simulink model "dcdctest"  (R2023b)
settings: Solver=VariableStepAuto  StartTime=0.0  StopTime=10  RelTol=1e-3
values from neighbouring files (symbols this model uses):
  cell_cap_Ah = 2.2    [find_maximum_ovlp.m]    (also in main.m)
  dst_q_cls = zeros(50, 2)    [main.m]
  dst_trg_soc_av = zeros(50, 1)    [main.m]
  soc = soc_in    [balance_costF.m]    (also in find_maximum_ovlp.m = fix(rand (1, cell_count) * 100); log_clustering.m; main.m = [39    39    20    72    81    92    51    11    60]; plot_final.m)
  src_q_cls = zeros(50, 2)    [main.m]
  src_trg_soc_av = zeros(50, 1)    [main.m]
undefined symbols (not defined in the file or in its folder): Ion, Lithium
libraries: spsIdealSwitchLib x18, spsBatteryLib x12, spsControlledCurrentSourceLib x8, spsVoltageMeasurementLib x8, simulink x4, slpidlib x3, spspowerguiLib x2
(part 2 of 2)

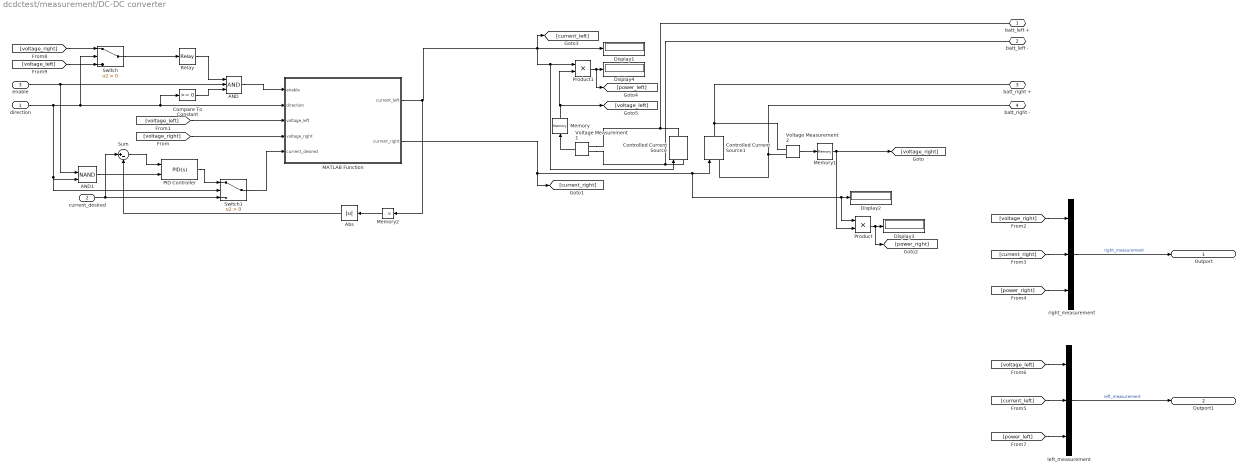
== system dcdctest/measurement/DC-DC converter ==
  direction : Inport
  current_desired : Inport  Port=2
  enable : Inport  Port=3
  AND : Logic  Inputs=3  IconShape=distinctive  AllPortsSameDT=off  OutDataTypeStr=boolean
  AND1 : Logic  Operator=NAND  IconShape=distinctive  AllPortsSameDT=off  OutDataTypeStr=boolean
  Abs : Abs  SaturateOnIntegerOverflow=off
  Compare To Constant : simulink/Logic and Bit Operations/Compare To Constant  relop=>=  const=0  OutDataTypeStr=boolean
  Controlled Current Source : spsControlledCurrentSourceLib/Controlled Current Source  Initialize=on  Source_Type=DC  Amplitude=0  Phase=0  Frequency=0  Measurements=None
  Controlled Current Source1 : spsControlledCurrentSourceLib/Controlled Current Source  Initialize=on  Source_Type=AC  Amplitude=0  Phase=0  Frequency=0  Measurements=None
  Display{1..4} (4 alike) : Display
  MATLAB Function : MATLAB Function  TreatAsAtomicUnit=on
  Memory : Memory
  Memory1 : Memory
  Memory2 : Memory
  PID Controller : slpidlib/PID Controller  Controller=PID  Form=Parallel  TimeDomain=Continuous-time  UseExternalTs=off  SampleTime=-1  IntegratorMethod=Forward Euler  FilterMethod=Forward Euler  ControllerParametersSource=internal  P=0.01  I=2  UseKiTs=off  D=0  N=100  UseFilter=on  TunerSelectOption=Transfer Function Based (PID Tuner App)  InitialConditionSource=internal  InitialConditionForIntegrator=0  InitialConditionForFilter=0  DifferentiatorICPrevScaledInput=0  ExternalReset=level  TrackingMode=off  Kt=1  LimitOutput=on  SatLimitsSource=internal  UpperSaturationLimit=2  LowerSaturationLimit=0  LinearizeAsGain=on  AntiWindupMode=none  Kb=1  LimitIntegrator=off  UpperIntegratorSaturationLimit=inf  LowerIntegratorSaturationLimit=-inf  POutMin=[]  POutMax=[]  IOutMin=[]  IOutMax=[]  DOutMin=[]  DOutMax=[]  NOutMin=[]  NOutMax=[]  SumOutMin=[]  SumOutMax=[]  SaturationOutMin=[]  SaturationOutMax=[]  PParamMin=[]  PParamMax=[]  IParamMin=[]  IParamMax=[]  DParamMin=[]  DParamMax=[]  NParamMin=[]  NParamMax=[]  KbParamMin=[]  KbParamMax=[]  KtParamMin=[]  KtParamMax=[]  KbOutMin=[]  KbOutMax=[]  KtOutMin=[]  KtOutMax=[]  IntegratorOutMin=[]  IntegratorOutMax=[]  FilterOutMin=[]  FilterOutMax=[]  SumI1OutMin=[]  SumI1OutMax=[]  SumI2OutMin=[]  SumI2OutMax=[]  SumI3OutMin=[]  SumI3OutMax=[]  SumI4OutMin=[]  SumI4OutMax=[]  SumDOutMin=[]  SumDOutMax=[]  DifferentiatorOutMin=[]  DifferentiatorOutMax=[]  FilterDiffOutCoefMin=[]  FilterDiffOutCoefMax=[]  ReciprocalOutMin=[]  ReciprocalOutMax=[]  SumDenOutMin=[]  SumDenOutMax=[]  SumNumOutMin=[]  SumNumOutMax=[]  DivideOutMin=[]  DivideOutMax=[]  UdiffTsProdOutMin=[]  UdiffTsProdOutMax=[]  NTsProdOutMin=[]  NTsProdOutMax=[]  UintegralTsProdOutMin=[]  UintegralTsProdOutMax=[]  UngainTsProdOutMin=[]  UngainTsProdOutMax=[]  ClampingZeroOutDataTypeStr=Inherit: Inherit via back propagation  ClampingZeroOutMin=[]  ClampingZeroOutMax=[]  FilterDenConstantOutDataTypeStr=Inherit: Inherit via back propagation  FilterDenConstantOutMin=[]  FilterDenConstantOutMax=[]  PCopyOutDataTypeStr=Inherit: Inherit via back propagation  PCopyOutMin=[]  PCopyOutMax=[]  NCopyOutDataTypeStr=Inherit: Inherit via back propagation  NCopyOutMin=[]  NCopyOutMax=[]  IntegratorContinuousStateAttributes=''  IntegratorStateMustResolveToSignalObject=off  IntegratorRTWStateStorageClass=Auto  FilterContinuousStateAttributes=''  FilterStateMustResolveToSignalObject=off  FilterRTWStateStorageClass=Auto  ParallelPVariant=InternalParameters  IdealPVariant=Disabled  IVariant=InternalParameters  DVariant=InternalParameters  IntegratorVariant=Continuous  SatVariant=Enabled  AWVariant=Passthrough  PCopyVariant=Disabled  TRVariant=Disabled  FdbkBlocksVariant=Forward  IdealPFdbkVariant=Disabled  SatFdbkVariant=Disabled  DerivativeFilterVariant=ContFilter  NVariant=InternalParameters  NCopyVariant=Disabled  FilterICVariant=InternalICsFilter  IntegratorICVariant=InternalICs  ExternalResetVariant=ExternalReset  TRSumVariant=Passthrough  SumFdbkVariant=Disabled  SumVariant=Sum_PID  TsampFilterVariant=InternalTs  TsampNgainVariant=Passthrough  TsampIntegralVariant=Disabled_SignalSpec  ExternalSaturationOutDataTypeStr=Inherit: Same as second input
  Product : Product
  Product1 : Product
  Relay : Relay  OnSwitchValue=3.5  OffSwitchValue=2
  Sum : Sum  Inputs=|+-
  Switch : Switch  Criteria=u2 > Threshold  SaturateOnIntegerOverflow=off  InputSameDT=off
  Switch1 : Switch  Criteria=u2 > Threshold  SaturateOnIntegerOverflow=off  InputSameDT=off
  Voltage Measurement1 : spsVoltageMeasurementLib/Voltage Measurement  PhasorSimulation=off  OutputType=Complex  PSBequivalent=0
  Voltage Measurement2 : spsVoltageMeasurementLib/Voltage Measurement  PhasorSimulation=off  OutputType=Complex  PSBequivalent=0
  left_measurement : Mux  Inputs=3
  right_measurement : Mux  Inputs=3
  batt_left + : PMIOPort  Side=Left
  batt_left - : PMIOPort  Port=2  Side=Left
  batt_right + : PMIOPort  Port=3  Side=Right
  batt_right - : PMIOPort  Port=4  Side=Right
  Outport : Outport
  Outport1 : Outport  Port=2
  wires:
  MATLAB Function/1(current_left) -> Memory2/1, Controlled Current Source/1, Product1/1, [current_left], Display1/1
  enable/1 -> AND1/1, AND/2
  Voltage Measurement2/1 -> Memory1/1
  direction/1 -> Compare To Constant/1, MATLAB Function/2(direction), Switch/2, AND1/2, Switch1/2
  [voltage_right] -> MATLAB Function/4(voltage_right)
  [voltage_left] -> MATLAB Function/3(voltage_left)
  Product/1 -> [power_right], Display3/1
  Product1/1 -> [power_left], Display4/1
  current_desired/1 -> Sum/1, Switch1/3
  [voltage_right] -> right_measurement/1
  [current_right] -> right_measurement/2
  [power_right] -> right_measurement/3
  [power_left] -> left_measurement/3
  [current_left] -> left_measurement/2
  [voltage_left] -> left_measurement/1
  right_measurement/1 -> Outport/1  "right_measurement"
  left_measurement/1 -> Outport1/1  "left_measurement"
  Voltage Measurement1/1 -> Memory/1
  Relay/1 -> AND/1
  AND/1 -> MATLAB Function/1(enable)
  Switch/1 -> Relay/1
  [voltage_left] -> Switch/3
  [voltage_right] -> Switch/1
  Memory/1 -> Product1/2, [voltage_left]
  Memory1/1 -> [voltage_right], Product/2
  Compare To Constant/1 -> AND/3
  Sum/1 -> PID Controller/1
  PID Controller/1 -> Switch1/1
  Switch1/1 -> MATLAB Function/5(current_desired)
  AND1/1 -> PID Controller/2
  Memory2/1 -> Abs/1
  MATLAB Function/2(current_right) -> [current_right], Product/1, Display2/1, Controlled Current Source1/1
  Abs/1 -> Sum/2
  connections:
  Voltage Measurement1/LConn1 -- batt_left +/RConn1 -- Controlled Current Source/RConn1
  Controlled Current Source1/RConn1 -- batt_right +/RConn1 -- Voltage Measurement2/LConn1
  Voltage Measurement2/LConn2 -- Controlled Current Source1/LConn1 -- batt_right -/RConn1
  Voltage Measurement1/LConn2 -- batt_left -/RConn1 -- Controlled Current Source/LConn1

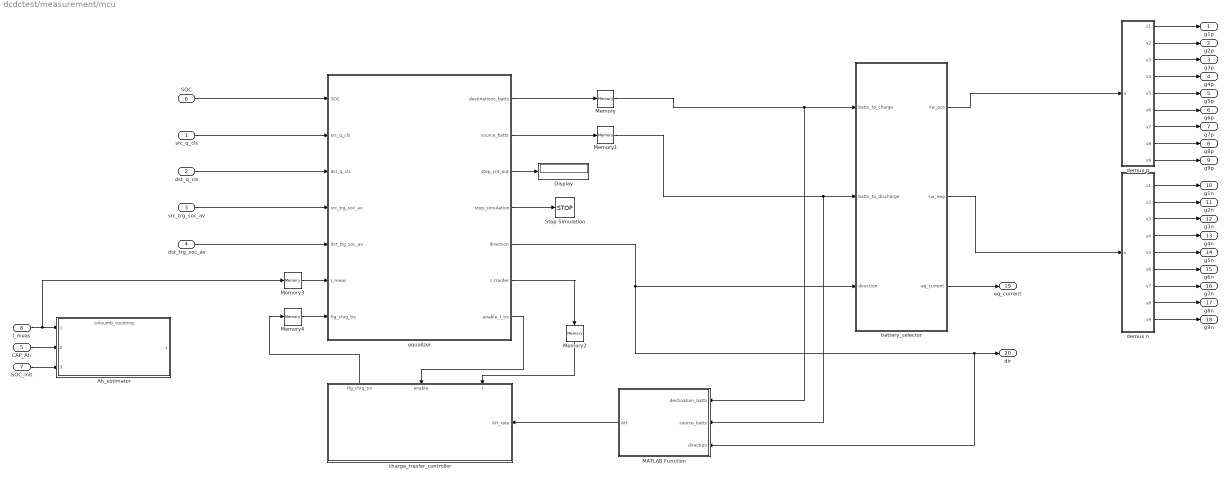
== system dcdctest/measurement/mcu ==
  src_q_cls : Inport
  dst_q_cls : Inport  Port=2
  src_trg_soc_av : Inport  Port=3
  dst_trg_soc_av : Inport  Port=4
  CAP_Ah : Inport  Port=5
  SOC : Inport  Port=6
  SOC_init : Inport  Port=7
  I_meas : Inport  Port=8
  Ah_estimator : ModelReference  ModelNameDialog=coloumb_counting.slx  SimulationMode=Normal  ModelReferenceVersion=1.13
  Display : Display
  MATLAB Function : MATLAB Function  TreatAsAtomicUnit=on
  Memory{,1..4} (5 alike) : Memory
  Stop Simulation : Stop
  battery_selector : MATLAB Function  TreatAsAtomicUnit=on
  charge_trasfer_controller : Subsystem
      settings: PortSchema="{\"entries\":[{\"content\":{\"sides\":[{\"content\":{},\"type\":\"ConnectorPlacement.EquallySpacedRectSide\",\"uuid\":\"48c70ec0-4261-4909-a719-c03e97c3e4ca\"},{\"content\":{\"connectorIds\":[\"In3\"],\"side\":\"RIGHT\"},\"type\":\"ConnectorPlacement.EquallySpacedRectSide\",\"uuid\":\"8a44a88a-c632-4005-90b8-1b0d09211c10\"},{\"content\":{\"connectorIds\":[\"Out1\",\"In1\",\"In2\"],\"side\":\"TOP\"},\"type\":\"ConnectorPlacement.EquallySpacedRectSide\",\"uuid\":\"71bafe47-820a-4a08-9919-e54bf550fba8\"}]},\"type\":\"ConnectorPlacement.EquallySpacedConnector\",\"uuid\":\"9c996bd2-099e-4131-a64b-67fbb4a72a45\"}],\"packageUris\":[\"http://schema.mathworks.com/mf0/Connector/R2020b\"],\"version\":\"1.0\"}"
  demux n : MATLAB Function  TreatAsAtomicUnit=on
  demux p : MATLAB Function  TreatAsAtomicUnit=on
  equalizer : MATLAB Function  TreatAsAtomicUnit=on
  g1p : Outport
  g2p : Outport  Port=2
  g3p : Outport  Port=3
  g4p : Outport  Port=4
  g5p : Outport  Port=5
  g6p : Outport  Port=6
  g7p : Outport  Port=7
  g8p : Outport  Port=8
  g9p : Outport  Port=9
  g1n : Outport  Port=10
  g2n : Outport  Port=11
  g3n : Outport  Port=12
  g4n : Outport  Port=13
  g5n : Outport  Port=14
  g6n : Outport  Port=15
  g7n : Outport  Port=16
  g8n : Outport  Port=17
  g9n : Outport  Port=18
  eq_current : Outport  Port=19
  dir : Outport  Port=20
  wires:
  battery_selector/3(eq_current) -> eq_current/1
  Memory/1 -> MATLAB Function/1(destination_batts), battery_selector/1(batts_to_charge)
  demux n/3(s3) -> g3n/1
  demux n/7(s7) -> g7n/1
  demux n/2(s2) -> g2n/1
  equalizer/1(destinations_batts) -> Memory/1
  dst_q_cls/1 -> equalizer/3(dst_q_cls)
  equalizer/4(stop_simulation) -> Stop Simulation/1
  demux p/7(s7) -> g7p/1
  Memory1/1 -> MATLAB Function/2(source_batts), battery_selector/2(batts_to_discharge)
  demux n/6(s6) -> g6n/1
  battery_selector/1(sw_pos) -> demux p/1(u)
  equalizer/2(source_batts) -> Memory1/1
  equalizer/3(step_cnt_out) -> Display/1
  battery_selector/2(sw_neg) -> demux n/1(u)
  src_q_cls/1 -> equalizer/2(src_q_cls)
  src_trg_soc_av/1 -> equalizer/4(src_trg_soc_av)
  demux n/5(s5) -> g5n/1
  demux n/8(s8) -> g8n/1
  dst_trg_soc_av/1 -> equalizer/5(dst_trg_soc_av)
  demux p/9(s9) -> g9p/1
  demux p/4(s4) -> g4p/1
  demux p/1(s1) -> g1p/1
  SOC/1 -> equalizer/1(SOC)
  demux p/5(s5) -> g5p/1
  demux p/2(s2) -> g2p/1
  demux p/8(s8) -> g8p/1
  demux n/1(s1) -> g1n/1
  demux n/4(s4) -> g4n/1
  demux n/9(s9) -> g9n/1
  demux p/3(s3) -> g3p/1
  demux p/6(s6) -> g6p/1
  SOC_init/1 -> Ah_estimator/3
  CAP_Ah/1 -> Ah_estimator/2
  MATLAB Function/1(AH) -> charge_trasfer_controller/3(AH_rate)
  equalizer/6(I_tranfer) -> Memory2/1
  equalizer/7(enable_I_trs) -> charge_trasfer_controller/1(enable)
  charge_trasfer_controller/1(flg_chrg_trs) -> Memory4/1
  equalizer/5(direction) -> MATLAB Function/3(direction), dir/1, battery_selector/3(direction)
  I_meas/1 -> Memory3/1, Ah_estimator/1
  Memory2/1 -> charge_trasfer_controller/2(I)
  Memory3/1 -> equalizer/6(I_meas)
  Memory4/1 -> equalizer/7(flg_chrg_trs)

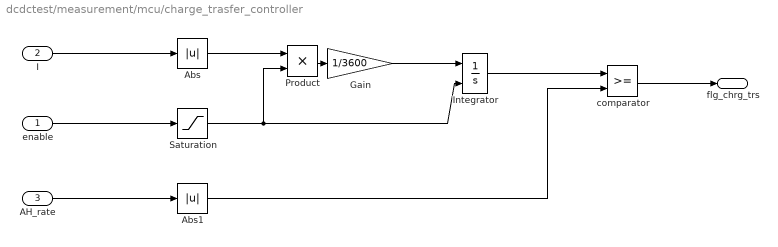
== system dcdctest/measurement/mcu/charge_trasfer_controller ==
  enable : Inport
  I : Inport  Port=2
  AH_rate : Inport  Port=3
  Abs : Abs  SaturateOnIntegerOverflow=off
  Abs1 : Abs  SaturateOnIntegerOverflow=off
  Gain : Gain  Gain=1/3600
  Integrator : Integrator  ExternalReset=either
  Product : Product
  Saturation : Saturate  UpperLimit=1  LowerLimit=0
  comparator : RelationalOperator  OutDataTypeStr=boolean  RndMeth=Simplest  InputSameDT=off
  flg_chrg_trs : Outport
  wires:
  comparator/1 -> flg_chrg_trs/1
  AH_rate/1 -> Abs1/1
  Abs/1 -> Product/1
  Integrator/1 -> comparator/1
  Product/1 -> Gain/1
  enable/1 -> Saturation/1
  Gain/1 -> Integrator/1
  Saturation/1 -> Product/2, Integrator/2
  I/1 -> Abs/1
  Abs1/1 -> comparator/2

== matlab function dcdctest/DC-DC converter2/MATLAB Function ==
  data: enable input; current_left output; direction input; voltage_left input; voltage_right input; current_right output; current_desired input
function [current_left, current_right] = current_controller(enable, direction, voltage_left, voltage_right, current_desired)    
    current_left = 0;
    current_right = 0;
if(enable)
    %% left side sink, right side source
    if(direction == 0) 
        % variables definition
        current_sink = -1 * current_desired;
        voltage_sink = voltage_left;
        voltage_source = voltage_right;
        power_source = 0;
        power_sink = 0;

        % input and output power must match
        power_sink = current_sink * voltage_sink;
        power_source = power_sink;
        if(voltage_source ~= 0)
            current_source =  -1 * (power_source / voltage_source);
        else
            current_source = -1 * current_sink;
        end
        % power delivery
        if(current_sink > 0)
            current_sink = current_sink * -1;
        end
        if(current_source < 0)
            current_source = current_source * -1;
        end
        current_left = current_sink;
        current_right = current_source;
    %% right side source, left side sink
    elseif(direction == 1)
        % variables definition
        current_sink = -1 * current_desired;
        voltage_sink = voltage_right;
        voltage_source = voltage_left;
        power_source = 0;
        power_sink = 0;

        % input and output power must match
        power_sink = current_sink * voltage_sink;
        power_source = power_sink;
        if(voltage_source ~= 0)
            current_source =  -1 * (power_source / voltage_source);
        else
            current_source = -1 * current_sink;
        end
        % power delivery
        current_left = current_source;
        current_right = current_sink;
    end

else
    current_left = 0;
    current_right = 0;
end
end

== matlab function dcdctest/mcu/equalizer ==
  data: destinations_batts output; SOC input; source_batts output [..50]; src_q_cls input; dst_q_cls input; src_trg_soc_av input; dst_trg_soc_av input; I_meas input; step_cnt_out output; stop_simulation output; direction output; I_tranfer output; enable_I_trs output; flg_chrg_trs input
function [destinations_batts, source_batts, step_cnt_out, stop_simulation, direction, I_tranfer, enable_I_trs] = battery_selector(SOC, src_q_cls, dst_q_cls, src_trg_soc_av, dst_trg_soc_av, I_meas, flg_chrg_trs)


I_tranfer  = 0;
stop_simulation  = 0;
source_batts = [0 0];
destinations_batts = [0 0];
dst_trg_soc_av_tmp = dst_trg_soc_av;
src_trg_soc_av_tmp = src_trg_soc_av;

dst_trg_soc_av_tmp(dst_trg_soc_av == 0) = Inf;
% src_trg_soc_av_tmp(src_trg_soc_av == 0) = Inf;
% the number of steps to equlalize the battery pack
step = length(src_q_cls);

persistent step_cnt;
persistent I_cells_source;
persistent I_cells_destination;
persistent dir;
persistent enable;



if isempty(step_cnt)
    step_cnt = 1;
    assert(1, 'Simulation terminated because x >= 10')

end

if isempty(I_cells_source)
    I_cells_source = 0;
end
if isempty(I_cells_destination)
    I_cells_destination = 0;
end
if isempty(dir)
    dir = -1;
end
if isempty(enable)
    enable = 0;
end



soc = SOC';
if src_q_cls(step_cnt, :) > 0


    source_batts = src_q_cls(step_cnt, :);
    I_cells_source = I_meas(source_batts(1, 1));       % source cells current
    destinations_batts = dst_q_cls(step_cnt, :);
    I_cells_destination = I_meas(destinations_batts(1, 1));  % destication cells current



    if(dir == -1 && flg_chrg_trs == 0) % dischaege source if in the begining of charge transfering
        I_tranfer = I_cells_source;
        enable = 1; % start counting coulombs
        dir = 0; 
    end
    if(dir == 0)
        I_tranfer = I_cells_source;
    end

    if(dir == 0 && flg_chrg_trs == 1 && enable == 1) % reset the flag
        enable = 0;
    end

    if(dir == 0 && flg_chrg_trs == 0 && enable == 0) % charge the destination if the prevoius charge transfer terminated
        I_tranfer = I_cells_destination;
        enable = 1;
        dir = 1;
    end
    if(dir == 1)
        I_tranfer = I_cells_destination;
    end

    if(dir == 1 && flg_chrg_trs == 1 && enable == 1) % reset the flag
        enable = 0;
    end

    if(dir == 1 && flg_chrg_trs == 0 && enable == 0) % charge transfer terminated
        dir = -1;
    end
    
    sm = mean(soc(src_q_cls(step_cnt, 1):src_q_cls(step_cnt, 2)));
    dm = mean(soc(dst_q_cls(step_cnt, 1):dst_q_cls(step_cnt, 2)));
    if(sm <= src_trg_soc_av_tmp(step_cnt) || dm >= dst_trg_soc_av_tmp(step_cnt)) && dir == -1
        step_cnt = step_cnt + 1;
    end
else
    direction = 0;
    I_cells_source = 0;
    I_cells_destination = 0;
    dir = -1;
    stop_simulation  = 1;
    enable = 0
end
direction = dir;
enable_I_trs = enable;


step_cnt_out = step_cnt;

end

== matlab function dcdctest/mcu1/battery_selector ==
  data: batts_to_charge input; sw_pos output; sw_neg output; batts_to_discharge input; direction input; eq_current output
function [sw_pos, sw_neg, eq_current] = battery_selector(batts_to_charge, batts_to_discharge, direction)
    sw_pos = 0;
    sw_neg = 0;
    eq_current = 0;
    eq_current_tmp = 0;
% to prevent invalid switch selection
if ( batts_to_charge(1, 1) <= batts_to_charge(1, 2) && ...
     batts_to_discharge(1, 1) <= batts_to_discharge(1, 2))
    
    % charge the capacitor using batteries
    if(direction == 0)
        sw_pos = batts_to_discharge(1, 1);
        sw_neg = batts_to_discharge(1, 2);
        eq_current_tmp = 2;        
    % charge the battery using capacitor
    elseif(direction == 1)
        sw_pos = batts_to_charge(1, 1);
        sw_neg = batts_to_charge(1, 2);
        eq_current_tmp = 2;
    else
        sw_pos = 0;
        sw_neg = 0;

    end


    eq_current = eq_current_tmp * 0.5;

end


end

== matlab function dcdctest/mcu1/demux n ==
  data: u input; s1 output; s2 output; s3 output; s4 output; s5 output; s6 output; s7 output; s8 output; s9 output
function [s1, s2, s3, s4, s5, s6, s7, s8, s9] = demux(u)

    switch(u)
        case 1
            s1 = 1; s2 = 0;	s3 = 0; s4 = 0; s5 = 0; s6 = 0; s7 = 0; s8 = 0; s9 = 0;
        case 2      	
            s1 = 0; s2 = 1;	s3 = 0; s4 = 0; s5 = 0; s6 = 0; s7 = 0; s8 = 0; s9 = 0;
        case 3      	
            s1 = 0; s2 = 0;	s3 = 1; s4 = 0; s5 = 0; s6 = 0; s7 = 0; s8 = 0; s9 = 0;
        case 4      	
            s1 = 0; s2 = 0;	s3 = 0; s4 = 1; s5 = 0; s6 = 0; s7 = 0; s8 = 0; s9 = 0;
        case 5      	
            s1 = 0; s2 = 0;	s3 = 0; s4 = 0; s5 = 1; s6 = 0; s7 = 0; s8 = 0; s9 = 0;
        case 6      	
            s1 = 0; s2 = 0;	s3 = 0; s4 = 0; s5 = 0; s6 = 1; s7 = 0; s8 = 0; s9 = 0;
        case 7      
            s1 = 0; s2 = 0;	s3 = 0; s4 = 0; s5 = 0; s6 = 0; s7 = 1; s8 = 0; s9 = 0;
        case 8      	
            s1 = 0; s2 = 0;	s3 = 0; s4 = 0; s5 = 0; s6 = 0; s7 = 0; s8 = 1; s9 = 0;
        case 9      
            s1 = 0; s2 = 0;	s3 = 0; s4 = 0; s5 = 0; s6 = 0; s7 = 0; s8 = 0; s9 = 1;
        otherwise   	
            s1 = 0; s2 = 0;	s3 = 0; s4 = 0; s5 = 0; s6 = 0; s7 = 0; s8 = 0; s9 = 0;
    end
end

== matlab function dcdctest/mcu1/demux p ==
  data: u input; s1 output; s2 output; s3 output; s4 output; s5 output; s6 output; s7 output; s8 output; s9 output
function [s1, s2, s3, s4, s5, s6, s7, s8, s9] = demux(u)

    switch(u)
        case 1
            s1 = 1; s2 = 0;	s3 = 0; s4 = 0; s5 = 0; s6 = 0; s7 = 0; s8 = 0; s9 = 0;
        case 2      	
            s1 = 0; s2 = 1;	s3 = 0; s4 = 0; s5 = 0; s6 = 0; s7 = 0; s8 = 0; s9 = 0;
        case 3      	
            s1 = 0; s2 = 0;	s3 = 1; s4 = 0; s5 = 0; s6 = 0; s7 = 0; s8 = 0; s9 = 0;
        case 4      	
            s1 = 0; s2 = 0;	s3 = 0; s4 = 1; s5 = 0; s6 = 0; s7 = 0; s8 = 0; s9 = 0;
        case 5      	
            s1 = 0; s2 = 0;	s3 = 0; s4 = 0; s5 = 1; s6 = 0; s7 = 0; s8 = 0; s9 = 0;
        case 6      	
            s1 = 0; s2 = 0;	s3 = 0; s4 = 0; s5 = 0; s6 = 1; s7 = 0; s8 = 0; s9 = 0;
        case 7      
            s1 = 0; s2 = 0;	s3 = 0; s4 = 0; s5 = 0; s6 = 0; s7 = 1; s8 = 0; s9 = 0;
        case 8      	
            s1 = 0; s2 = 0;	s3 = 0; s4 = 0; s5 = 0; s6 = 0; s7 = 0; s8 = 1; s9 = 0;
        case 9      
            s1 = 0; s2 = 0;	s3 = 0; s4 = 0; s5 = 0; s6 = 0; s7 = 0; s8 = 0; s9 = 1;
        otherwise   	
            s1 = 0; s2 = 0;	s3 = 0; s4 = 0; s5 = 0; s6 = 0; s7 = 0; s8 = 0; s9 = 0;
    end
end

== matlab function dcdctest/mcu1/equalizer ==
  data: destinations_batts output; SOC input; source_batts output [..50]; src_q_cls input; dst_q_cls input; src_trg_soc_av input; dst_trg_soc_av input; I_meas input; step_cnt_out output; stop_simulation output; direction output; I_tranfer output; enable_I_trs output; flg_chrg_trs input
function [destinations_batts, source_batts, step_cnt_out, stop_simulation, direction, I_tranfer, enable_I_trs] = battery_selector(SOC, src_q_cls, dst_q_cls, src_trg_soc_av, dst_trg_soc_av, I_meas, flg_chrg_trs)


I_tranfer  = 0;
stop_simulation  = 0;
source_batts = [0 0];
destinations_batts = [0 0];
dst_trg_soc_av_tmp = dst_trg_soc_av;
src_trg_soc_av_tmp = src_trg_soc_av;

dst_trg_soc_av_tmp(dst_trg_soc_av == 0) = Inf;
% src_trg_soc_av_tmp(src_trg_soc_av == 0) = Inf;
% the number of steps to equlalize the battery pack
step = length(src_q_cls);

persistent step_cnt;
persistent I_cells_source;
persistent I_cells_destination;
persistent dir;
persistent enable;



if isempty(step_cnt)
    step_cnt = 1;
    assert(1, 'Simulation terminated because x >= 10')

end

if isempty(I_cells_source)
    I_cells_source = 0;
end
if isempty(I_cells_destination)
    I_cells_destination = 0;
end
if isempty(dir)
    dir = -1;
end
if isempty(enable)
    enable = 0;
end



soc = SOC';
if src_q_cls(step_cnt, :) > 0


    source_batts = src_q_cls(step_cnt, :);
    I_cells_source = I_meas(source_batts(1, 1));       % source cells current
    destinations_batts = dst_q_cls(step_cnt, :);
    I_cells_destination = I_meas(destinations_batts(1, 1));  % destication cells current



    if(dir == -1 && flg_chrg_trs == 0) % dischaege source if in the begining of charge transfering
        I_tranfer = I_cells_source;
        enable = 1; % start counting coulombs
        dir = 0; 
    end
    if(dir == 0)
        I_tranfer = I_cells_source;
    end

    if(dir == 0 && flg_chrg_trs == 1 && enable == 1) % reset the flag
        enable = 0;
    end

    if(dir == 0 && flg_chrg_trs == 0 && enable == 0) % charge the destination if the prevoius charge transfer terminated
        I_tranfer = I_cells_destination;
        enable = 1;
        dir = 1;
    end
    if(dir == 1)
        I_tranfer = I_cells_destination;
    end

    if(dir == 1 && flg_chrg_trs == 1 && enable == 1) % reset the flag
        enable = 0;
    end

    if(dir == 1 && flg_chrg_trs == 0 && enable == 0) % charge transfer terminated
        dir = -1;
    end
    
    sm = mean(soc(src_q_cls(step_cnt, 1):src_q_cls(step_cnt, 2)));
    dm = mean(soc(dst_q_cls(step_cnt, 1):dst_q_cls(step_cnt, 2)));
    if(sm <= src_trg_soc_av_tmp(step_cnt) || dm >= dst_trg_soc_av_tmp(step_cnt)) && dir == -1
        step_cnt = step_cnt + 1;
    end
else
    direction = 0;
    I_cells_source = 0;
    I_cells_destination = 0;
    dir = -1;
    stop_simulation  = 1;
    enable = 0
end
direction = dir;
enable_I_trs = enable;


step_cnt_out = step_cnt;

end

== matlab function dcdctest/measurement/DC-DC converter/MATLAB Function ==
  data: enable input; current_left output; direction input; voltage_left input; voltage_right input; current_right output; current_desired input
function [current_left, current_right] = current_controller(enable, direction, voltage_left, voltage_right, current_desired)    
    current_left = 0;
    current_right = 0;
if(enable)
    %% left side sink, right side source
    if(direction == 0) 
        % variables definition
        current_sink = -1 * current_desired;
        voltage_sink = voltage_left;
        voltage_source = voltage_right;
        power_source = 0;
        power_sink = 0;

        % input and output power must match
        power_sink = current_sink * voltage_sink;
        power_source = power_sink;
        if(voltage_source ~= 0)
            current_source =  -1 * (power_source / voltage_source);
        else
            current_source = -1 * current_sink;
        end
        % power delivery
        if(current_sink > 0)
            current_sink = current_sink * -1;
        end
        if(current_source < 0)
            current_source = current_source * -1;
        end
        current_left = current_sink;
        current_right = current_source;
    %% left side source, right side sink
    elseif(direction == 1)
        % variables definition
        current_sink = -1 * current_desired;
        voltage_sink = voltage_right;
        voltage_source = voltage_left;
        power_source = 0;
        power_sink = 0;

        % input and output power must match
        power_sink = current_sink * voltage_sink;
        power_source = power_sink;
        if(voltage_source ~= 0)
            current_source =  -1 * (power_source / voltage_source);
        else
            current_source = -1 * current_sink;
        end
        % power delivery
        current_left = current_source;
        current_right = current_sink;
    end

else
    current_left = 0;
    current_right = 0;
end
end

== matlab function dcdctest/measurement/mcu/MATLAB Function ==
  data: destination_batts input; AH output; source_batts input; direction input
function AH = fcn(destination_batts, source_batts, direction)
AH_Base = 0.001;
AH = AH_Base;
source_batts_number = source_batts(1,2) - source_batts(1,1) + 1;
destination_batts_number = destination_batts(1,2) - destination_batts(1,1) + 1;


if source_batts_number > destination_batts_number && direction == 0 % draw less current from source 
    AH = destination_batts_number / source_batts_number * AH_Base;
elseif source_batts_number < destination_batts_number && direction == 1 % inject less current to destination
    AH = source_batts_number / destination_batts_number * AH_Base;
else 
    AH = AH_Base;
end

== matlab function dcdctest/measurement/mcu/battery_selector ==
  data: batts_to_charge input; sw_pos output; sw_neg output; batts_to_discharge input; direction input; eq_current output
function [sw_pos, sw_neg, eq_current] = battery_selector(batts_to_charge, batts_to_discharge, direction)
    sw_pos = 0;
    sw_neg = 0;
    eq_current = 0;
    eq_current_tmp = 0;
% to prevent invalid switch selection
if ( batts_to_charge(1, 1) <= batts_to_charge(1, 2) && ...
     batts_to_discharge(1, 1) <= batts_to_discharge(1, 2))
    
    % charge the capacitor using batteries
    if(direction == 0)
        sw_pos = batts_to_discharge(1, 1);
        sw_neg = batts_to_discharge(1, 2);
        eq_current_tmp = 2;        
    % charge the battery using capacitor
    elseif(direction == 1)
        sw_pos = batts_to_charge(1, 1);
        sw_neg = batts_to_charge(1, 2);
        eq_current_tmp = 2;
    else
        sw_pos = 0;
        sw_neg = 0;

    end


    eq_current = eq_current_tmp * 0.5;

end


end

== matlab function dcdctest/measurement/mcu/demux n ==
  data: u input; s1 output; s2 output; s3 output; s4 output; s5 output; s6 output; s7 output; s8 output; s9 output
function [s1, s2, s3, s4, s5, s6, s7, s8, s9] = demux(u)

    switch(u)
        case 1
            s1 = 1; s2 = 0;	s3 = 0; s4 = 0; s5 = 0; s6 = 0; s7 = 0; s8 = 0; s9 = 0;
        case 2      	
            s1 = 0; s2 = 1;	s3 = 0; s4 = 0; s5 = 0; s6 = 0; s7 = 0; s8 = 0; s9 = 0;
        case 3      	
            s1 = 0; s2 = 0;	s3 = 1; s4 = 0; s5 = 0; s6 = 0; s7 = 0; s8 = 0; s9 = 0;
        case 4      	
            s1 = 0; s2 = 0;	s3 = 0; s4 = 1; s5 = 0; s6 = 0; s7 = 0; s8 = 0; s9 = 0;
        case 5      	
            s1 = 0; s2 = 0;	s3 = 0; s4 = 0; s5 = 1; s6 = 0; s7 = 0; s8 = 0; s9 = 0;
        case 6      	
            s1 = 0; s2 = 0;	s3 = 0; s4 = 0; s5 = 0; s6 = 1; s7 = 0; s8 = 0; s9 = 0;
        case 7      
            s1 = 0; s2 = 0;	s3 = 0; s4 = 0; s5 = 0; s6 = 0; s7 = 1; s8 = 0; s9 = 0;
        case 8      	
            s1 = 0; s2 = 0;	s3 = 0; s4 = 0; s5 = 0; s6 = 0; s7 = 0; s8 = 1; s9 = 0;
        case 9      
            s1 = 0; s2 = 0;	s3 = 0; s4 = 0; s5 = 0; s6 = 0; s7 = 0; s8 = 0; s9 = 1;
        otherwise   	
            s1 = 0; s2 = 0;	s3 = 0; s4 = 0; s5 = 0; s6 = 0; s7 = 0; s8 = 0; s9 = 0;
    end
end

== matlab function dcdctest/measurement/mcu/demux p ==
  data: u input; s1 output; s2 output; s3 output; s4 output; s5 output; s6 output; s7 output; s8 output; s9 output
function [s1, s2, s3, s4, s5, s6, s7, s8, s9] = demux(u)

    switch(u)
        case 1
            s1 = 1; s2 = 0;	s3 = 0; s4 = 0; s5 = 0; s6 = 0; s7 = 0; s8 = 0; s9 = 0;
        case 2      	
            s1 = 0; s2 = 1;	s3 = 0; s4 = 0; s5 = 0; s6 = 0; s7 = 0; s8 = 0; s9 = 0;
        case 3      	
            s1 = 0; s2 = 0;	s3 = 1; s4 = 0; s5 = 0; s6 = 0; s7 = 0; s8 = 0; s9 = 0;
        case 4      	
            s1 = 0; s2 = 0;	s3 = 0; s4 = 1; s5 = 0; s6 = 0; s7 = 0; s8 = 0; s9 = 0;
        case 5      	
            s1 = 0; s2 = 0;	s3 = 0; s4 = 0; s5 = 1; s6 = 0; s7 = 0; s8 = 0; s9 = 0;
        case 6      	
            s1 = 0; s2 = 0;	s3 = 0; s4 = 0; s5 = 0; s6 = 1; s7 = 0; s8 = 0; s9 = 0;
        case 7      
            s1 = 0; s2 = 0;	s3 = 0; s4 = 0; s5 = 0; s6 = 0; s7 = 1; s8 = 0; s9 = 0;
        case 8      	
            s1 = 0; s2 = 0;	s3 = 0; s4 = 0; s5 = 0; s6 = 0; s7 = 0; s8 = 1; s9 = 0;
        case 9      
            s1 = 0; s2 = 0;	s3 = 0; s4 = 0; s5 = 0; s6 = 0; s7 = 0; s8 = 0; s9 = 1;
        otherwise   	
            s1 = 0; s2 = 0;	s3 = 0; s4 = 0; s5 = 0; s6 = 0; s7 = 0; s8 = 0; s9 = 0;
    end
end

== matlab function dcdctest/measurement/mcu/equalizer ==
  data: destinations_batts output; SOC input; source_batts output [..50]; src_q_cls input; dst_q_cls input; src_trg_soc_av input; dst_trg_soc_av input; I_meas input; step_cnt_out output; stop_simulation output; direction output; I_tranfer output; enable_I_trs output; flg_chrg_trs input
function [destinations_batts, source_batts, step_cnt_out, stop_simulation, direction, I_tranfer, enable_I_trs] = battery_selector(SOC, src_q_cls, dst_q_cls, src_trg_soc_av, dst_trg_soc_av, I_meas, flg_chrg_trs)


I_tranfer  = 0;
stop_simulation  = 0;
source_batts = [0 0];
destinations_batts = [0 0];
dst_trg_soc_av_tmp = dst_trg_soc_av;
src_trg_soc_av_tmp = src_trg_soc_av;

dst_trg_soc_av_tmp(dst_trg_soc_av == 0) = Inf;
% src_trg_soc_av_tmp(src_trg_soc_av == 0) = Inf;
% the number of steps to equlalize the battery pack
step = length(src_q_cls);

persistent step_cnt;
persistent I_cells_source;
persistent I_cells_destination;
persistent dir;
persistent enable;



if isempty(step_cnt)
    step_cnt = 1;
    assert(1, 'Simulation terminated because x >= 10')

end

if isempty(I_cells_source)
    I_cells_source = 0;
end
if isempty(I_cells_destination)
    I_cells_destination = 0;
end
if isempty(dir)
    dir = -1;
end
if isempty(enable)
    enable = 0;
end



soc = SOC';
if src_q_cls(step_cnt, :) > 0


    source_batts = src_q_cls(step_cnt, :);
    I_cells_source = I_meas(source_batts(1, 1));       % source cells current
    destinations_batts = dst_q_cls(step_cnt, :);
    I_cells_destination = I_meas(destinations_batts(1, 1));  % destication cells current



    if(dir == -1 && flg_chrg_trs == 0) % dischaege source if in the begining of charge transfering
        I_tranfer = I_cells_source;
        enable = 1; % start counting coulombs
        dir = 0; 
    end
    if(dir == 0)
        I_tranfer = I_cells_source;
    end

    if(dir == 0 && flg_chrg_trs == 1 && enable == 1) % reset the flag
        enable = 0;
    end

    if(dir == 0 && flg_chrg_trs == 0 && enable == 0) % charge the destination if the prevoius charge transfer terminated
        I_tranfer = I_cells_destination;
        enable = 1;
        dir = 1;
    end
    if(dir == 1)
        I_tranfer = I_cells_destination;
    end

    if(dir == 1 && flg_chrg_trs == 1 && enable == 1) % reset the flag
        enable = 0;
    end

    if(dir == 1 && flg_chrg_trs == 0 && enable == 0) % charge transfer terminated
        dir = -1;
    end
    
    sm = mean(soc(src_q_cls(step_cnt, 1):src_q_cls(step_cnt, 2)));
    dm = mean(soc(dst_q_cls(step_cnt, 1):dst_q_cls(step_cnt, 2)));
    if(sm <= src_trg_soc_av_tmp(step_cnt) || dm >= dst_trg_soc_av_tmp(step_cnt)) && dir == -1
        step_cnt = step_cnt + 1;
    end
else
    direction = 0;
    I_cells_source = 0;
    I_cells_destination = 0;
    dir = -1;
    stop_simulation  = 1;
    enable = 0
end
direction = dir;
enable_I_trs = enable;


step_cnt_out = step_cnt;

end

== matlab function dcdctest/DC-DC converter1/MATLAB Function ==
  data: enable input; current_left output; direction input; voltage_left input; voltage_right input; current_right output; current_desired input
function [current_left, current_right] = current_controller(enable, direction, voltage_left, voltage_right, current_desired)    
    current_left = 0;
    current_right = 0;
if(enable)
    %% left side sink, right side source
    if(direction == 0) 
        % variables definition
        current_sink = -1 * current_desired;
        voltage_sink = voltage_left;
        voltage_source = voltage_right;
        power_source = 0;
        power_sink = 0;

        % input and output power must match
        power_sink = current_sink * voltage_sink;
        power_source = power_sink;
        if(voltage_source ~= 0)
            current_source =  -1 * (power_source / voltage_source);
        else
            current_source = -1 * current_sink;
        end
        % power delivery
        if(current_sink > 0)
            current_sink = current_sink * -1;
        end
        if(current_source < 0)
            current_source = current_source * -1;
        end
        current_left = current_sink;
        current_right = current_source;
    %% left side source, right side sink
    elseif(direction == 1)
        % variables definition
        current_sink = -1 * current_desired;
        voltage_sink = voltage_right;
        voltage_source = voltage_left;
        power_source = 0;
        power_sink = 0;

        % input and output power must match
        power_sink = current_sink * voltage_sink;
        power_source = power_sink;
        if(voltage_source ~= 0)
            current_source =  -1 * (power_source / voltage_source);
        else
            current_source = -1 * current_sink;
        end
        % power delivery
        current_left = current_source;
        current_right = current_sink;
    end

else
    current_left = 0;
    current_right = 0;
end
end

== matlab function dcdctest/DC-DC converter/MATLAB Function ==
  data: enable input; current_left output; direction input; voltage_left input; voltage_right input; current_right output; current_desired input
function [current_left, current_right] = current_controller(enable, direction, voltage_left, voltage_right, current_desired)    
    current_left = 0;
    current_right = 0;
if(enable)
    %% left side sink, right side source
    if(direction == 0) 
        % variables definition
        current_sink = -1 * current_desired;
        voltage_sink = voltage_left;
        voltage_source = voltage_right;
        power_source = 0;
        power_sink = 0;

        % input and output power must match
        power_sink = current_sink * voltage_sink;
        power_source = power_sink;
        if(voltage_source ~= 0)
            current_source =  -1 * (power_source / voltage_source);
        else
            current_source = -1 * current_sink;
        end
        % power delivery
        if(current_sink > 0)
            current_sink = current_sink * -1;
        end
        if(current_source < 0)
            current_source = current_source * -1;
        end
        current_left = current_sink;
        current_right = current_source;
    %% left side source, right side sink
    elseif(direction == 1)
        % variables definition
        current_sink = -1 * current_desired;
        voltage_sink = voltage_right;
        voltage_source = voltage_left;
        power_source = 0;
        power_sink = 0;

        % input and output power must match
        power_sink = current_sink * voltage_sink;
        power_source = power_sink;
        if(voltage_source ~= 0)
            current_source =  -1 * (power_source / voltage_source);
        else
            current_source = -1 * current_sink;
        end
        % power delivery
        current_left = current_source;
        current_right = current_sink;
    end

else
    current_left = 0;
    current_right = 0;
end
end

== matlab function dcdctest/mcu/battery_selector ==
  data: batts_to_charge input; sw_pos output; sw_neg output; batts_to_discharge input; direction input; eq_current output
function [sw_pos, sw_neg, eq_current] = battery_selector(batts_to_charge, batts_to_discharge, direction)
    sw_pos = 0;
    sw_neg = 0;
    eq_current = 0;
    eq_current_tmp = 0;
% to prevent invalid switch selection
if ( batts_to_charge(1, 1) <= batts_to_charge(1, 2) && ...
     batts_to_discharge(1, 1) <= batts_to_discharge(1, 2))
    
    % charge the capacitor using batteries
    if(direction == 0)
        sw_pos = batts_to_discharge(1, 1);
        sw_neg = batts_to_discharge(1, 2);
        eq_current_tmp = 2;        
    % charge the battery using capacitor
    elseif(direction == 1)
        sw_pos = batts_to_charge(1, 1);
        sw_neg = batts_to_charge(1, 2);
        eq_current_tmp = 2;
    else
        sw_pos = 0;
        sw_neg = 0;

    end


    eq_current = eq_current_tmp * 0.5;

end


end

== matlab function dcdctest/mcu/demux n ==
  data: u input; s1 output; s2 output; s3 output; s4 output; s5 output; s6 output; s7 output; s8 output; s9 output
function [s1, s2, s3, s4, s5, s6, s7, s8, s9] = demux(u)

    switch(u)
        case 1
            s1 = 1; s2 = 0;	s3 = 0; s4 = 0; s5 = 0; s6 = 0; s7 = 0; s8 = 0; s9 = 0;
        case 2      	
            s1 = 0; s2 = 1;	s3 = 0; s4 = 0; s5 = 0; s6 = 0; s7 = 0; s8 = 0; s9 = 0;
        case 3      	
            s1 = 0; s2 = 0;	s3 = 1; s4 = 0; s5 = 0; s6 = 0; s7 = 0; s8 = 0; s9 = 0;
        case 4      	
            s1 = 0; s2 = 0;	s3 = 0; s4 = 1; s5 = 0; s6 = 0; s7 = 0; s8 = 0; s9 = 0;
        case 5      	
            s1 = 0; s2 = 0;	s3 = 0; s4 = 0; s5 = 1; s6 = 0; s7 = 0; s8 = 0; s9 = 0;
        case 6      	
            s1 = 0; s2 = 0;	s3 = 0; s4 = 0; s5 = 0; s6 = 1; s7 = 0; s8 = 0; s9 = 0;
        case 7      
            s1 = 0; s2 = 0;	s3 = 0; s4 = 0; s5 = 0; s6 = 0; s7 = 1; s8 = 0; s9 = 0;
        case 8      	
            s1 = 0; s2 = 0;	s3 = 0; s4 = 0; s5 = 0; s6 = 0; s7 = 0; s8 = 1; s9 = 0;
        case 9      
            s1 = 0; s2 = 0;	s3 = 0; s4 = 0; s5 = 0; s6 = 0; s7 = 0; s8 = 0; s9 = 1;
        otherwise   	
            s1 = 0; s2 = 0;	s3 = 0; s4 = 0; s5 = 0; s6 = 0; s7 = 0; s8 = 0; s9 = 0;
    end
end

== matlab function dcdctest/mcu/MATLAB Function ==
  data: destination_batts input; AH output; source_batts input; direction input
function AH = fcn(destination_batts, source_batts, direction)
AH_Base = 0.001;
AH = AH_Base;
source_batts_number = source_batts(1,2) - source_batts(1,1) + 1;
destination_batts_number = destination_batts(1,2) - destination_batts(1,1) + 1;


if source_batts_number > destination_batts_number && direction == 0 % draw less current from source 
    AH = destination_batts_number / source_batts_number * AH_Base;
elseif source_batts_number < destination_batts_number && direction == 1 % inject less current to destination
    AH = source_batts_number / destination_batts_number * AH_Base;
else 
    AH = AH_Base;
end

== matlab function dcdctest/mcu/demux p ==
  data: u input; s1 output; s2 output; s3 output; s4 output; s5 output; s6 output; s7 output; s8 output; s9 output
function [s1, s2, s3, s4, s5, s6, s7, s8, s9] = demux(u)

    switch(u)
        case 1
            s1 = 1; s2 = 0;	s3 = 0; s4 = 0; s5 = 0; s6 = 0; s7 = 0; s8 = 0; s9 = 0;
        case 2      	
            s1 = 0; s2 = 1;	s3 = 0; s4 = 0; s5 = 0; s6 = 0; s7 = 0; s8 = 0; s9 = 0;
        case 3      	
            s1 = 0; s2 = 0;	s3 = 1; s4 = 0; s5 = 0; s6 = 0; s7 = 0; s8 = 0; s9 = 0;
        case 4      	
            s1 = 0; s2 = 0;	s3 = 0; s4 = 1; s5 = 0; s6 = 0; s7 = 0; s8 = 0; s9 = 0;
        case 5      	
            s1 = 0; s2 = 0;	s3 = 0; s4 = 0; s5 = 1; s6 = 0; s7 = 0; s8 = 0; s9 = 0;
        case 6      	
            s1 = 0; s2 = 0;	s3 = 0; s4 = 0; s5 = 0; s6 = 1; s7 = 0; s8 = 0; s9 = 0;
        case 7      
            s1 = 0; s2 = 0;	s3 = 0; s4 = 0; s5 = 0; s6 = 0; s7 = 1; s8 = 0; s9 = 0;
        case 8      	
            s1 = 0; s2 = 0;	s3 = 0; s4 = 0; s5 = 0; s6 = 0; s7 = 0; s8 = 1; s9 = 0;
        case 9      
            s1 = 0; s2 = 0;	s3 = 0; s4 = 0; s5 = 0; s6 = 0; s7 = 0; s8 = 0; s9 = 1;
        otherwise   	
            s1 = 0; s2 = 0;	s3 = 0; s4 = 0; s5 = 0; s6 = 0; s7 = 0; s8 = 0; s9 = 0;
    end
end
